simulink model "flightgear"  (Simulink 7.8)
settings: Solver=ode45  StartTime=0.0  StopTime=10.0  RelTol=1e-3
libraries: aerolibfltsims x2, aerolibanimutils x1
settings Model: Creator=Dan  LastModifiedBy=Dan

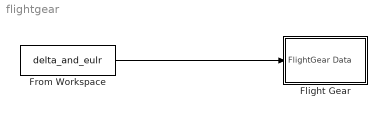
== system flightgear ==
  Flight Gear : Subsystem
  From Workspace : FromWorkspace  VariableName=delta_and_eulr  SampleTime=0
  wires:
  From Workspace/1 -> Flight Gear/1(FlightGear Data)

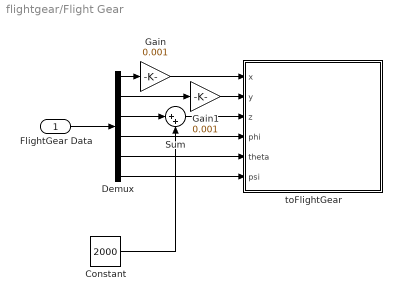
== system flightgear/Flight Gear ==
  FlightGear Data : Inport
  Constant : Constant  Value=2000
  Demux : Demux  Outputs=6
  Gain : Gain  Gain=0.001
  Gain1 : Gain  Gain=0.001
  Sum : Sum  Inputs=|++
  toFlightGear : Subsystem  TreatAsAtomicUnit=on
  wires:
  Demux/1 -> Gain/1
  Demux/2 -> Gain1/1
  Demux/4 -> toFlightGear/4(phi)
  Demux/5 -> toFlightGear/5(theta)
  Demux/6 -> toFlightGear/6(psi)
  FlightGear Data/1 -> Demux/1
  Demux/3 -> Sum/1
  Sum/1 -> toFlightGear/3(z)
  Constant/1 -> Sum/2
  Gain/1 -> toFlightGear/1(x)
  Gain1/1 -> toFlightGear/2(y)

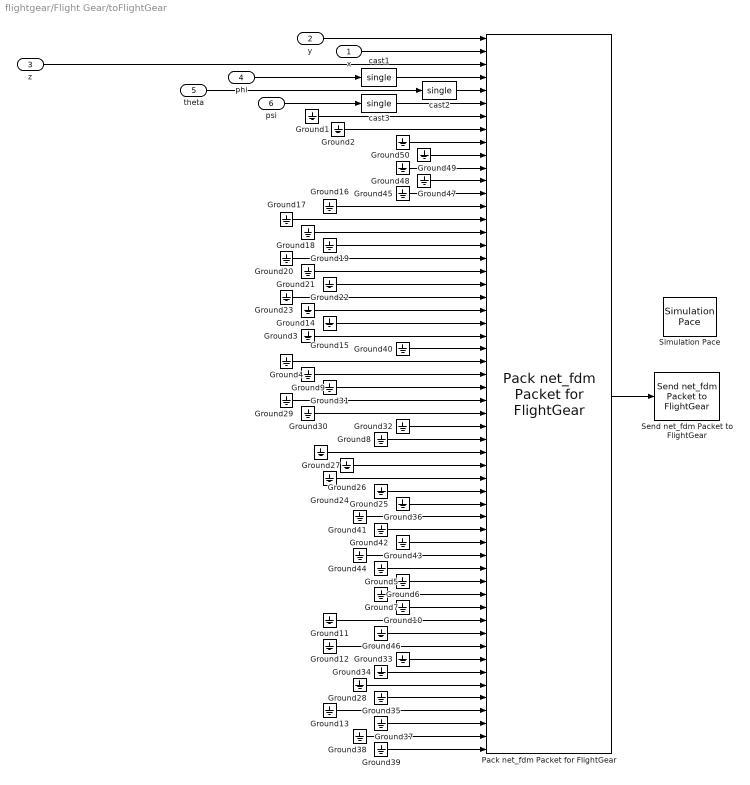
== system flightgear/Flight Gear/toFlightGear ==
  x : Inport
  y : Inport  Port=2
  z : Inport  Port=3
  phi : Inport  Port=4
  theta : Inport  Port=5
  psi : Inport  Port=6
  Ground{1..50} (50 alike) : Ground
  Pack net_fdm Packet for FlightGear : aerolibfltsims/Pack net_fdm Packet for FlightGear  FlightGearVersion=v2.0  ShowPositionAttitudeInputs=on  ShowVelocityAccelerationInputs=on  ShowControlSurfacePositionInputs=on  ShowEngineFuelInputs=on  ShowLandingGearInputs=on  ShowEnvironmentInputs=on  SampleTime=1/30
      settings: AttributesFormatString=FG VERSION: %<FlightGearVersion>
  Send net_fdm Packet to FlightGear : aerolibfltsims/Send net_fdm Packet to FlightGear  DestinationIpAddress=127.0.0.1  DestinationPort=5502  LocalIpPort=-1  varLen=off  SampleTime=1/30
  Simulation Pace : aerolibanimutils/Simulation Pace  SimulationPace=1  SleepMode=MATLAB Thread  OutputPaceError=off  SampleTime=0.001
      settings: AttributesFormatString=%<SimulationPace> sec/sec
  cast1 : DataTypeConversion  OutDataTypeStr=single  SaturateOnIntegerOverflow=on
  cast2 : DataTypeConversion  OutDataTypeStr=single  SaturateOnIntegerOverflow=on
  cast3 : DataTypeConversion  OutDataTypeStr=single  SaturateOnIntegerOverflow=on
  wires:
  Ground16/1 -> Pack net_fdm Packet for FlightGear/14
  Ground17/1 -> Pack net_fdm Packet for FlightGear/15
  Ground18/1 -> Pack net_fdm Packet for FlightGear/16
  Ground19/1 -> Pack net_fdm Packet for FlightGear/17
  Ground20/1 -> Pack net_fdm Packet for FlightGear/18
  Ground21/1 -> Pack net_fdm Packet for FlightGear/19
  Ground22/1 -> Pack net_fdm Packet for FlightGear/20
  Ground23/1 -> Pack net_fdm Packet for FlightGear/21
  Ground14/1 -> Pack net_fdm Packet for FlightGear/22
  Ground15/1 -> Pack net_fdm Packet for FlightGear/23
  Ground24/1 -> Pack net_fdm Packet for FlightGear/35
  Ground25/1 -> Pack net_fdm Packet for FlightGear/36
  Ground36/1 -> Pack net_fdm Packet for FlightGear/37
  Ground41/1 -> Pack net_fdm Packet for FlightGear/38
  Ground42/1 -> Pack net_fdm Packet for FlightGear/39
  Ground43/1 -> Pack net_fdm Packet for FlightGear/40
  Ground44/1 -> Pack net_fdm Packet for FlightGear/41
  Ground11/1 -> Pack net_fdm Packet for FlightGear/46
  Ground46/1 -> Pack net_fdm Packet for FlightGear/47
  Ground12/1 -> Pack net_fdm Packet for FlightGear/48
  Ground28/1 -> Pack net_fdm Packet for FlightGear/51
  Ground13/1 -> Pack net_fdm Packet for FlightGear/53
  Ground1/1 -> Pack net_fdm Packet for FlightGear/7
  Ground2/1 -> Pack net_fdm Packet for FlightGear/8
  Ground3/1 -> Pack net_fdm Packet for FlightGear/24
  Ground5/1 -> Pack net_fdm Packet for FlightGear/42
  Ground6/1 -> Pack net_fdm Packet for FlightGear/43
  Ground7/1 -> Pack net_fdm Packet for FlightGear/44
  Ground4/1 -> Pack net_fdm Packet for FlightGear/26
  Ground8/1 -> Pack net_fdm Packet for FlightGear/32
  Pack net_fdm Packet for FlightGear/1 -> Send net_fdm Packet to FlightGear/1
  Ground10/1 -> Pack net_fdm Packet for FlightGear/45
  Ground9/1 -> Pack net_fdm Packet for FlightGear/27
  Ground27/1 -> Pack net_fdm Packet for FlightGear/33
  Ground26/1 -> Pack net_fdm Packet for FlightGear/34
  Ground29/1 -> Pack net_fdm Packet for FlightGear/29
  Ground30/1 -> Pack net_fdm Packet for FlightGear/30
  Ground31/1 -> Pack net_fdm Packet for FlightGear/28
  Ground32/1 -> Pack net_fdm Packet for FlightGear/31
  Ground33/1 -> Pack net_fdm Packet for FlightGear/49
  Ground34/1 -> Pack net_fdm Packet for FlightGear/50
  Ground35/1 -> Pack net_fdm Packet for FlightGear/52
  Ground37/1 -> Pack net_fdm Packet for FlightGear/54
  Ground38/1 -> Pack net_fdm Packet for FlightGear/55
  Ground39/1 -> Pack net_fdm Packet for FlightGear/56
  Ground40/1 -> Pack net_fdm Packet for FlightGear/25
  Ground45/1 -> Pack net_fdm Packet for FlightGear/13
  Ground47/1 -> Pack net_fdm Packet for FlightGear/12
  Ground48/1 -> Pack net_fdm Packet for FlightGear/11
  Ground49/1 -> Pack net_fdm Packet for FlightGear/10
  Ground50/1 -> Pack net_fdm Packet for FlightGear/9
  phi/1 -> cast1/1
  psi/1 -> cast3/1
  cast1/1 -> Pack net_fdm Packet for FlightGear/4
  cast2/1 -> Pack net_fdm Packet for FlightGear/5
  cast3/1 -> Pack net_fdm Packet for FlightGear/6
  theta/1 -> cast2/1
  z/1 -> Pack net_fdm Packet for FlightGear/3
  y/1 -> Pack net_fdm Packet for FlightGear/1
  x/1 -> Pack net_fdm Packet for FlightGear/2
